simulink model "exercise_2_2"  (R2017a)
settings: Solver=ode1  StartTime=0.0  StopTime=SimulationTime  FixedStep=0.001  RelTol=1e-3
values from neighbouring files (symbols this model uses):
  d_gain = 4.4384e+01    (= 44.384)    [exercise_2.m]
  m = 1    [exercise_2.m]
  p_gain = 2.7887e+03    (= 2788.7)    [exercise_2.m]
libraries: simulink x1
settings Model: Creator=marce  LastModifiedBy=marce

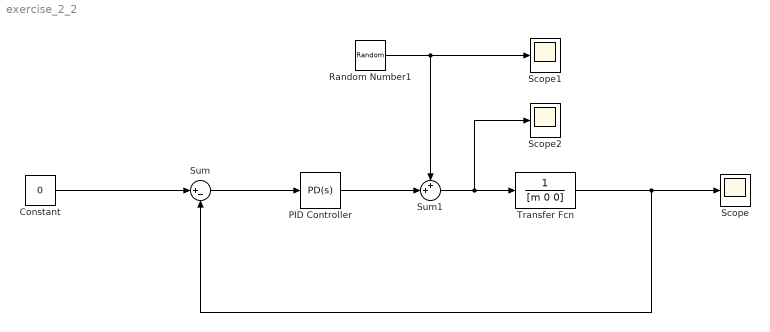
== system exercise_2_2 ==
  Constant : Constant  Value=0
  PID Controller : simulink/Continuous/PID Controller  Controller=PD  TimeDomain=Continuous-time  SampleTime=-1  IntegratorMethod=Forward Euler  FilterMethod=Forward Euler  Form=Parallel  UseFilter=on  ControllerParametersSource=internal  P=p_gain  I=0  D=d_gain  N=1000  InitialConditionSource=internal  InitialConditionForIntegrator=0  InitialConditionForFilter=0  ExternalReset=none  LimitOutput=off  UpperSaturationLimit=inf  LowerSaturationLimit=-inf  LinearizeAsGain=on  AntiWindupMode=none  Kb=1  TrackingMode=off  Kt=1  PParamMin=[]  PParamMax=[]  IParamMin=[]  IParamMax=[]  DParamMin=[]  DParamMax=[]  NParamMin=[]  NParamMax=[]  KbParamMin=[]  KbParamMax=[]  KtParamMin=[]  KtParamMax=[]  POutMin=[]  POutMax=[]  IOutMin=[]  IOutMax=[]  DOutMin=[]  DOutMax=[]  NOutMin=[]  NOutMax=[]  KbOutMin=[]  KbOutMax=[]  KtOutMin=[]  KtOutMax=[]  IntegratorOutMin=[]  IntegratorOutMax=[]  FilterOutMin=[]  FilterOutMax=[]  SumOutMin=[]  SumOutMax=[]  SumI1OutMin=[]  SumI1OutMax=[]  SumI2OutMin=[]  SumI2OutMax=[]  SumI3OutMin=[]  SumI3OutMax=[]  SumDOutMin=[]  SumDOutMax=[]  SaturationOutMin=[]  SaturationOutMax=[]  IntegratorContinuousStateAttributes=''  IntegratorStateMustResolveToSignalObject=off  IntegratorRTWStateStorageClass=Auto  FilterContinuousStateAttributes=''  FilterStateMustResolveToSignalObject=off  FilterRTWStateStorageClass=Auto  DifferentiatorICPrevScaledInput=0  DifferentiatorOutMin=[]  DifferentiatorOutMax=[]  InitialConditionSetting=State (most efficient)
  Random Number1 : RandomNumber  SampleTime=0.001
  Scope : Scope
  Scope1 : Scope
  Scope2 : Scope
  Sum : Sum  Inputs=|+-
  Sum1 : Sum  Inputs=++|
  Transfer Fcn : TransferFcn  Denominator=[m 0 0]
  wires:
  Sum1/1 -> Scope2/1, Transfer Fcn/1
  PID Controller/1 -> Sum1/2
  Sum/1 -> PID Controller/1
  Random Number1/1 -> Sum1/1, Scope1/1
  Constant/1 -> Sum/1
  Transfer Fcn/1 -> Sum/2, Scope/1
